simulink model "Lightning_McSeas_VCU_Current_Mode"  (R2021b)
settings: Solver=FixedStepDiscrete  StartTime=0.0  StopTime=10.0  FixedStep=0.01  RelTol=1e-3  EnableMultiTasking=on
PreLoadFcn:
  | try, model_open; catch, disp('Error occurred while executing model pre-load callback: model_open.m'); disp('Please assure that the MATLAB working directory is set to the model directory before opening.'); end
InitFcn:
  | try, model_open; catch, end
undefined symbols (not defined in the file): dataName, enumName, enumValue, GCM, raptor_get_safe_string
libraries: Raptor_lib x72, simulink x8
(part 3 of 3)

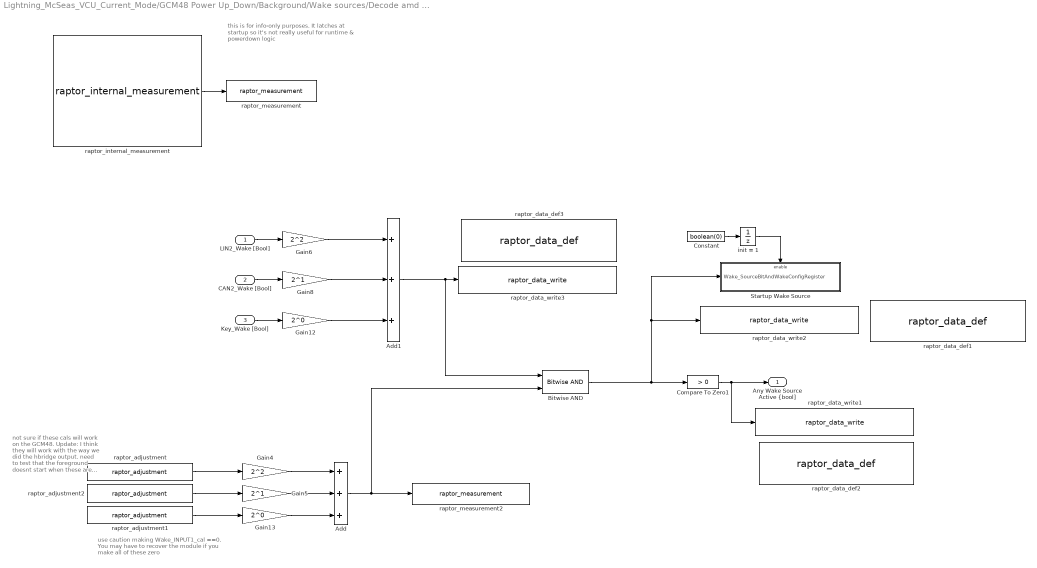
== system Lightning_McSeas_VCU_Current_Mode/GCM48 Power Up_Down/Background/Wake sources/Decode amd Ignore Some Wake Sources ==
  note: this is for info-only purposes. It latches at startup so it's not really useful for runtime & powerdown logic
  note: not sure if these cals will work on the GCM48. Update: I think they will work with the way we did the hbridge output. need to test that the foreground doesnt start when these are zero
  note: use caution making Wake_INPUT1_cal ==0. You may have to recover the module if you make all of these zero
  LIN2_Wake [Bool] : Inport
  CAN2_Wake [Bool] : Inport  Port=2
  Key_Wake [Bool] : Inport  Port=3
  Add : Sum  Inputs=3  OutDataTypeStr=uint16
  Add1 : Sum  Inputs=3  OutDataTypeStr=uint16
  Bitwise AND : simulink/Logic and Bit Operations/Bitwise Operator  logicop=AND  UseBitMask=off  NumInputPorts=2  BitMask=bin2dec('11011001')  BitMaskRealWorld=Stored Integer
  Compare To Zero1 : simulink/Logic and Bit Operations/Compare To Zero  relop=>  OutDataTypeStr=boolean
  Constant : Constant  Value=boolean(0)
  Gain12 : Gain  Gain=2^0  OutDataTypeStr=uint16
  Gain13 : Gain  Gain=2^0  OutDataTypeStr=uint16
  Gain4 : Gain  Gain=2^2  OutDataTypeStr=uint16
  Gain5 : Gain  Gain=2^1  OutDataTypeStr=uint16
  Gain6 : Gain  Gain=2^2  OutDataTypeStr=uint16
  Gain8 : Gain  Gain=2^1  OutDataTypeStr=uint16
  Startup Wake Source : Subsystem  TreatAsAtomicUnit=on
  init = 1 : UnitDelay  InitialCondition=1  SampleTime=-1  HasFrameUpgradeWarning=on
  raptor_adjustment : Raptor_lib/Data Storage/raptor_adjustment  paramName='GCM48Wake_LIN2_cal'  nameSource=Parameter  initValue=0  dataType=boolean  storage=Calibration  calDispType=Number  calEnum={'False', 'True'}  calGain=1.0  calOffset=0.0  calMax=inf  calMin=-inf  calFormat='-1'  calUnit='bool'  calHelp='1 configures the module to wake via this input, 0 ignores this input'  calAccess=4  calFunction=group  calDispHeaders=off  calColHeaders={'Col1' 'Col2' 'Col3'}  calRowHeaders={'Row1' 'Row2' 'Row3'}
      settings: SourceProductName=Raptor
  raptor_adjustment1 : Raptor_lib/Data Storage/raptor_adjustment  paramName='GCM48Wake_INPUT1_cal'  nameSource=Parameter  initValue=1  dataType=boolean  storage=Calibration  calDispType=Number  calEnum={'False', 'True'}  calGain=1.0  calOffset=0.0  calMax=inf  calMin=-inf  calFormat='-1'  calUnit='bool'  calHelp='1 configures the module to wake via this input, 0 ignores this input'  calAccess=4  calFunction=group  calDispHeaders=off  calColHeaders={'Col1' 'Col2' 'Col3'}  calRowHeaders={'Row1' 'Row2' 'Row3'}
      settings: SourceProductName=Raptor
  raptor_adjustment2 : Raptor_lib/Data Storage/raptor_adjustment  paramName='GCM48Wake_CAN2_cal'  nameSource=Parameter  initValue=0  dataType=boolean  storage=Calibration  calDispType=Number  calEnum={'False', 'True'}  calGain=1.0  calOffset=0.0  calMax=inf  calMin=-inf  calFormat='-1'  calUnit='bool'  calHelp='1 configures the module to wake via this input, 0 ignores this input'  calAccess=4  calFunction=group  calDispHeaders=off  calColHeaders={'Col1' 'Col2' 'Col3'}  calRowHeaders={'Row1' 'Row2' 'Row3'}
      settings: SourceProductName=Raptor
  raptor_data_def1 : Raptor_lib/Data Storage/raptor_data_def  dataName='Wake_SourceBitAndWakeConfigRegister'  initValue=0  dataType=uint16  storage=Volatile (RAM)  calVisible=on  calType=Measurement  calDispType=Number  calEnum={'False', 'True'}  calGain=1.0  calOffset=0  calMin=-inf  calMax=inf  calFormat='-1'  calUnit=''  calHelp=''  calAccess=2  calFunction=group  calDispHeaders=off  calColHeaders={'Col1' 'Col2' 'Col3'}  calRowHeaders={'Row1' 'Row2' 'Row3'}
      settings: SourceProductName=Raptor
  raptor_data_def2 : Raptor_lib/Data Storage/raptor_data_def  dataName='Wake_AnyWakeSourceActive'  initValue=0  dataType=boolean  storage=Volatile (RAM)  calVisible=on  calType=Measurement  calDispType=Number  calEnum={'False', 'True'}  calGain=1.0  calOffset=0  calMin=-inf  calMax=inf  calFormat='-1'  calUnit='any wake source is keeping the module alive'  calHelp='bool'  calAccess=2  calFunction=group  calDispHeaders=off  calColHeaders={'Col1' 'Col2' 'Col3'}  calRowHeaders={'Row1' 'Row2' 'Row3'}
      settings: SourceProductName=Raptor
  raptor_data_def3 : Raptor_lib/Data Storage/raptor_data_def  dataName='WakeSource_Current'  initValue=0  dataType=uint16  storage=Volatile (RAM)  calVisible=on  calType=Measurement  calDispType=Number  calEnum={'False', 'True'}  calGain=1.0  calOffset=0  calMin=-inf  calMax=inf  calFormat='-1'  calUnit='wake source at the current instant'  calHelp=''  calAccess=2  calFunction=group  calDispHeaders=off  calColHeaders={'Col1' 'Col2' 'Col3'}  calRowHeaders={'Row1' 'Row2' 'Row3'}
      settings: SourceProductName=Raptor
  raptor_data_write1 : Raptor_lib/Data Storage/raptor_data_write  dataName='Wake_AnyWakeSourceActive'  dataShape=Scalar  idxSource=Input Port  idxRow=1  idxCol=1
      settings: SourceProductName=Raptor
  raptor_data_write2 : Raptor_lib/Data Storage/raptor_data_write  dataName='Wake_SourceBitAndWakeConfigRegister'  dataShape=Scalar  idxSource=Input Port  idxRow=1  idxCol=1
      settings: SourceProductName=Raptor
  raptor_data_write3 : Raptor_lib/Data Storage/raptor_data_write  dataName='WakeSource_Current'  dataShape=Scalar  idxSource=Input Port  idxRow=1  idxCol=1
      settings: SourceProductName=Raptor
  raptor_internal_measurement : Raptor_lib/Input & Output/raptor_internal_measurement  resourceValues=OUTPUT1_VFB|OUTPUT2_VFB|OUTPUT3_VFB|OUTPUT4_VFB|OUTPUT5_VFB|OUTPUT6_VFB|OUTPUT7_VFB|OUTPUT8_VFB|OUTPUT11_VFB|OUTPUT12_VFB|OUTPUT13_VFB|OUTPUT14_VFB|OUTPUT15_VFB|OUTPUT2_DFB|OUTPUT3_DFB|HBRIDGE9_10_DFB|OUTPUT2_IFB|OUTPUT3_IFB|HBRIDGE9_10_IFB|SENS_SUPPLY1_VFB|SENS_SUPPLY2_VFB|NTC_TEMP|WAKE_SOURCE|(None)  resource=WAKE_SOURCE  out_eng=0  soft_filter=1  out_bool=0
      settings: SourceProductName=Raptor
  raptor_measurement : Raptor_lib/Data Storage/raptor_measurement  paramName='WakeSource_RaptorIntrnlMeas'  nameSource=Parameter  calDispType=Number  calEnum={'False', 'True'}  calGain=1.0  calOffset=0.0  calMax=inf  calMin=-inf  calFormat='-1'  calUnit='wake source at startup... kinda. it often reads that LIN work the module even if the LIN bus isnt connected.'  calHelp=''  calAccess=4  calFunction=group  calVisible=on
      settings: SourceProductName=Raptor
  raptor_measurement2 : Raptor_lib/Data Storage/raptor_measurement  paramName='WakeConfigRegister'  nameSource=Parameter  calDispType=Number  calEnum={'False', 'True'}  calGain=1.0  calOffset=0.0  calMax=inf  calMin=-inf  calFormat='-1'  calUnit='register'  calHelp=''  calAccess=4  calFunction=group  calVisible=on
      settings: SourceProductName=Raptor
  "Any Wake Source Active {bool]" : Outport  VectorParamsAs1DForOutWhenUnconnected=off
  wires:
  Key_Wake [Bool]/1 -> Gain12/1
  init = 1/1 -> Startup Wake Source/Enable
  Constant/1 -> init = 1/1
  Compare To Zero1/1 -> "Any Wake Source Active {bool]"/1, raptor_data_write1/1
  LIN2_Wake [Bool]/1 -> Gain6/1
  CAN2_Wake [Bool]/1 -> Gain8/1
  raptor_adjustment1/1 -> Gain13/1
  Gain13/1 -> Add/3
  Gain12/1 -> Add1/3
  Add1/1 -> raptor_data_write3/1, Bitwise AND/1
  Gain6/1 -> Add1/1
  Gain8/1 -> Add1/2
  Bitwise AND/1 -> raptor_data_write2/1, Startup Wake Source/1(Wake_SourceBitAndWakeConfigRegister), Compare To Zero1/1
  raptor_adjustment2/1 -> Gain5/1
  Gain5/1 -> Add/2
  Add/1 -> raptor_measurement2/1, Bitwise AND/2
  raptor_internal_measurement/1 -> raptor_measurement/1
  raptor_adjustment/1 -> Gain4/1
  Gain4/1 -> Add/1

== system Lightning_McSeas_VCU_Current_Mode/GCM48 Power Up_Down/Background/Wake sources/Dtc ==
  In : Inport
  Delay Input1 : UnitDelay  Description=Store in Global RAM  DisableCoverage=on  InitialCondition=init  SampleTime=-1  HasFrameUpgradeWarning=on
  Relational Operator : RelationalOperator  Operator===  OutDataTypeStr=boolean  RndMeth=Nearest  InputSameDT=on
  Bool : Outport  InitialOutput=0  VectorParamsAs1DForOutWhenUnconnected=off
  wires:
  In/1 -> Delay Input1/1, Relational Operator/1
  Delay Input1/1 -> Relational Operator/2
  Relational Operator/1 -> Bool/1

== system Lightning_McSeas_VCU_Current_Mode/GCM48 Power Up_Down/Background/Wake sources/Dtc1 ==
  In : Inport
  Delay Input1 : UnitDelay  Description=Store in Global RAM  DisableCoverage=on  InitialCondition=init  SampleTime=-1  HasFrameUpgradeWarning=on
  Relational Operator : RelationalOperator  Operator===  OutDataTypeStr=boolean  RndMeth=Nearest  InputSameDT=on
  Bool : Outport  InitialOutput=0  VectorParamsAs1DForOutWhenUnconnected=off
  wires:
  Relational Operator/1 -> Bool/1
  Delay Input1/1 -> Relational Operator/2
  In/1 -> Relational Operator/1, Delay Input1/1

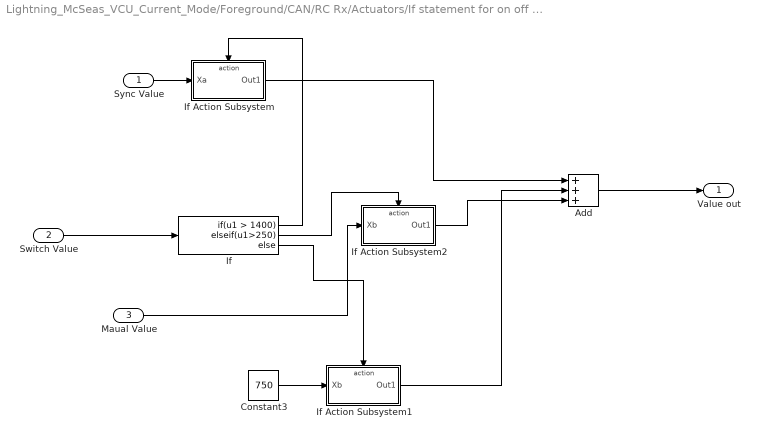
== system Lightning_McSeas_VCU_Current_Mode/Foreground/CAN/RC Rx/Actuators/If statement for on off switch1 ==
  Sync Value : Inport
  Switch Value : Inport  Port=2
  Maual Value : Inport  Port=3
  Add : Sum  Inputs=+++
  Constant3 : Constant  Value=750
  If : If  IfExpression=u1 > 1400  ElseIfExpressions=u1>250
  If Action Subsystem : Subsystem  TreatAsAtomicUnit=on
  If Action Subsystem1 : Subsystem  TreatAsAtomicUnit=on
  If Action Subsystem2 : Subsystem  TreatAsAtomicUnit=on
  Value out : Outport
  wires:
  If/3 -> If Action Subsystem1/Action
  Switch Value/1 -> If/1
  Sync Value/1 -> If Action Subsystem/1(Xa)
  If Action Subsystem1/1(Out1) -> Add/2
  Add/1 -> Value out/1
  If/1 -> If Action Subsystem/Action
  Constant3/1 -> If Action Subsystem1/1(Xb)
  If Action Subsystem/1(Out1) -> Add/1
  If/2 -> If Action Subsystem2/Action
  If Action Subsystem2/1(Out1) -> Add/3
  Maual Value/1 -> If Action Subsystem2/1(Xb)

== system Lightning_McSeas_VCU_Current_Mode/Foreground/CAN/RC Rx/Actuators/Subsystem ==
  Front left : Inport
  Rise of Front : Inport  Port=2
  Gain : Gain  Gain=1/1500
  Product : Product
  Actuator value : Outport
  wires:
  Front left/1 -> Gain/1
  Rise of Front/1 -> Product/1
  Gain/1 -> Product/2
  Product/1 -> Actuator value/1

== system Lightning_McSeas_VCU_Current_Mode/Foreground/CAN/RC Rx/Battery Charging/Max Voltage Cell Control ==
  note: 0 = Charging
      | 1 = STOP
  In1 : Inport
  Constant : Constant  Value=0
  Constant1 : Constant
  If : If  IfExpression=u1 > 4.15
  If Action Subsystem : Subsystem  TreatAsAtomicUnit=on
  If Action Subsystem1 : Subsystem  TreatAsAtomicUnit=on
  Merge : Merge
  Out1 : Outport
  wires:
  In1/1 -> If/1
  If/1 -> If Action Subsystem/Action
  If/2 -> If Action Subsystem1/Action
  Constant/1 -> If Action Subsystem/1(In1)
  Constant1/1 -> If Action Subsystem1/1(In1)
  If Action Subsystem/1(Out1) -> Merge/1
  If Action Subsystem1/1(Out1) -> Merge/2
  Merge/1 -> Out1/1

== system Lightning_McSeas_VCU_Current_Mode/Foreground/CAN/RC Rx/Battery Charging/Subsystem1 ==
  In1 : Inport
  In2 : Inport  Port=2
  Constant : Constant  Value=16
  Constant1 : Constant  Value=3.9
  If : If  IfExpression=u1 < 4.05  ElseIfExpressions=u1 < 4.10
  If Action Subsystem : Subsystem  TreatAsAtomicUnit=on
  If Action Subsystem1 : Subsystem  TreatAsAtomicUnit=on
  If Action Subsystem2 : Subsystem  TreatAsAtomicUnit=on
  Merge : Merge  Inputs=3
  Out1 : Outport
  wires:
  In1/1 -> If/1
  If/1 -> If Action Subsystem/Action
  If/3 -> If Action Subsystem1/Action
  Constant/1 -> If Action Subsystem/1(In1)
  Constant1/1 -> If Action Subsystem1/1(In1)
  If Action Subsystem/1(Out1) -> Merge/1
  If Action Subsystem1/1(Out1) -> Merge/3
  Merge/1 -> Out1/1
  If/2 -> If Action Subsystem2/Action
  In2/1 -> If Action Subsystem2/1(In1)
  If Action Subsystem2/1(Out1) -> Merge/2

== system Lightning_McSeas_VCU_Current_Mode/Foreground/CAN/RC Rx/Battery Charging/Switch Control ==
  note: 0 = Charging
      | 1 = STOP
  In1 : Inport
  Constant : Constant  Value=0
  Constant1 : Constant
  If : If  IfExpression=u1 > 1200
  If Action Subsystem : Subsystem  TreatAsAtomicUnit=on
  If Action Subsystem1 : Subsystem  TreatAsAtomicUnit=on
  Merge : Merge
  Out1 : Outport
  wires:
  In1/1 -> If/1
  If/1 -> If Action Subsystem/Action
  If/2 -> If Action Subsystem1/Action
  Constant/1 -> If Action Subsystem/1(In1)
  Constant1/1 -> If Action Subsystem1/1(In1)
  If Action Subsystem/1(Out1) -> Merge/1
  If Action Subsystem1/1(Out1) -> Merge/2
  Merge/1 -> Out1/1

== system Lightning_McSeas_VCU_Current_Mode/Foreground/CAN/RC Rx/Battery Switch/If statement for on off switch ==
  value in : Inport
  Constant2 : Constant
  Constant3 : Constant  Value=0
  If : If  IfExpression=u1 > 1200
  If Action Subsystem : Subsystem  TreatAsAtomicUnit=on
  If Action Subsystem1 : Subsystem  TreatAsAtomicUnit=on
  Merge : Merge
  Value out : Outport
  wires:
  If/2 -> If Action Subsystem1/Action
  value in/1 -> If/1
  Constant2/1 -> If Action Subsystem/1(Xa)
  If Action Subsystem1/1(Out1) -> Merge/2
  Merge/1 -> Value out/1
  If/1 -> If Action Subsystem/Action
  Constant3/1 -> If Action Subsystem1/1(Xb)
  If Action Subsystem/1(Out1) -> Merge/1

== system Lightning_McSeas_VCU_Current_Mode/Foreground/CAN/RC Rx/Battery Switch/If statement for on off switch1 ==
  value in : Inport
  Constant2 : Constant  OutDataTypeStr=boolean
  Constant3 : Constant  Value=0  OutDataTypeStr=boolean
  If : If  IfExpression=u1 > 1200
  If Action Subsystem : Subsystem  TreatAsAtomicUnit=on
  If Action Subsystem1 : Subsystem  TreatAsAtomicUnit=on
  Merge : Merge
  Value out : Outport
  wires:
  value in/1 -> If/1
  Constant2/1 -> If Action Subsystem/1(Xa)
  If Action Subsystem1/1(Out1) -> Merge/2
  Merge/1 -> Value out/1
  If/1 -> If Action Subsystem/Action
  Constant3/1 -> If Action Subsystem1/1(Xb)
  If Action Subsystem/1(Out1) -> Merge/1
  If/2 -> If Action Subsystem1/Action

== system Lightning_McSeas_VCU_Current_Mode/Foreground/CAN/RC Rx/Battery Switch/If statement for on off switch2 ==
  value in : Inport
  Constant2 : Constant
  Constant3 : Constant  Value=0
  If : If  IfExpression=u1 > 250
  If Action Subsystem : Subsystem  TreatAsAtomicUnit=on
  If Action Subsystem1 : Subsystem  TreatAsAtomicUnit=on
  Merge : Merge
  Value out : Outport
  wires:
  If/2 -> If Action Subsystem1/Action
  value in/1 -> If/1
  Constant2/1 -> If Action Subsystem/1(Xa)
  If Action Subsystem1/1(Out1) -> Merge/2
  Merge/1 -> Value out/1
  If/1 -> If Action Subsystem/Action
  Constant3/1 -> If Action Subsystem1/1(Xb)
  If Action Subsystem/1(Out1) -> Merge/1

== system Lightning_McSeas_VCU_Current_Mode/Foreground/CAN/RC Rx/MCU/If statement for on off switch1 ==
  value in : Inport
  Constant2 : Constant
  Constant3 : Constant  Value=0
  If : If  IfExpression=u1 > 1200
  If Action Subsystem : Subsystem  TreatAsAtomicUnit=on
  If Action Subsystem1 : Subsystem  TreatAsAtomicUnit=on
  Merge : Merge
  Value out : Outport
  wires:
  value in/1 -> If/1
  Constant2/1 -> If Action Subsystem/1(Xa)
  If Action Subsystem1/1(Out1) -> Merge/2
  Merge/1 -> Value out/1
  If/1 -> If Action Subsystem/Action
  Constant3/1 -> If Action Subsystem1/1(Xb)
  If Action Subsystem/1(Out1) -> Merge/1
  If/2 -> If Action Subsystem1/Action

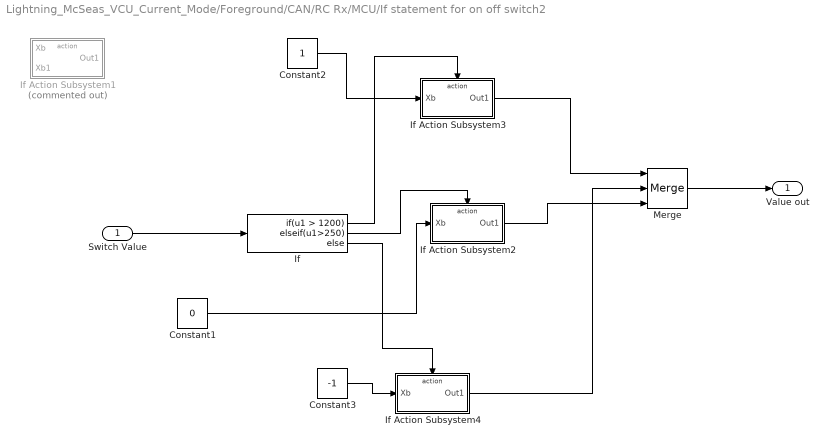
== system Lightning_McSeas_VCU_Current_Mode/Foreground/CAN/RC Rx/MCU/If statement for on off switch2 ==
  Switch Value : Inport
  Constant1 : Constant  Value=0
  Constant2 : Constant
  Constant3 : Constant  Value=-1
  If : If  IfExpression=u1 > 1200  ElseIfExpressions=u1>250
  If Action Subsystem1 : Subsystem  Commented=on  TreatAsAtomicUnit=on
  If Action Subsystem2 : Subsystem  TreatAsAtomicUnit=on
  If Action Subsystem3 : Subsystem  TreatAsAtomicUnit=on
  If Action Subsystem4 : Subsystem  TreatAsAtomicUnit=on
  Merge : Merge  Inputs=3
  Value out : Outport
  wires:
  If/3 -> If Action Subsystem4/Action
  Switch Value/1 -> If/1
  If Action Subsystem4/1(Out1) -> Merge/2
  Merge/1 -> Value out/1
  Constant3/1 -> If Action Subsystem4/1(Xb)
  If/2 -> If Action Subsystem2/Action
  If Action Subsystem2/1(Out1) -> Merge/3
  Constant1/1 -> If Action Subsystem2/1(Xb)
  Constant2/1 -> If Action Subsystem3/1(Xb)
  If Action Subsystem3/1(Out1) -> Merge/1
  If/1 -> If Action Subsystem3/Action

== system Lightning_McSeas_VCU_Current_Mode/Foreground/CAN/RC Rx/MCU/If statement for on off switch3 ==
  Switch Value : Inport
  Add : Sum  Inputs=+++
  Constant1 : Constant  Value=0
  Constant2 : Constant
  Constant3 : Constant  Value=-1
  If : If  IfExpression=u1 > 1200  ElseIfExpressions=u1>250
  If Action Subsystem1 : Subsystem  TreatAsAtomicUnit=on
  If Action Subsystem2 : Subsystem  TreatAsAtomicUnit=on
  If Action Subsystem3 : Subsystem  TreatAsAtomicUnit=on
  Value out : Outport
  wires:
  If/3 -> If Action Subsystem1/Action
  Switch Value/1 -> If Action Subsystem1/1(Xb), If Action Subsystem3/1(Xb), If/1
  If Action Subsystem1/1(Out1) -> Add/2
  Add/1 -> Value out/1
  Constant3/1 -> If Action Subsystem1/2(Xb1)
  If/2 -> If Action Subsystem2/Action
  If Action Subsystem2/1(Out1) -> Add/3
  Constant1/1 -> If Action Subsystem2/1(Xb)
  If/1 -> If Action Subsystem3/Action
  Constant2/1 -> If Action Subsystem3/2(Xb1)
  If Action Subsystem3/1(Out1) -> Add/1

== system Lightning_McSeas_VCU_Current_Mode/Foreground/CAN/RC Rx/MCU/If statement for on off switch4 ==
  value in : Inport
  Constant2 : Constant
  Constant3 : Constant  Value=0
  If : If  IfExpression=u1 >250
  If Action Subsystem : Subsystem  TreatAsAtomicUnit=on
  If Action Subsystem1 : Subsystem  TreatAsAtomicUnit=on
  Merge : Merge
  Value out : Outport
  wires:
  value in/1 -> If/1
  Constant2/1 -> If Action Subsystem/1(Xa)
  If Action Subsystem1/1(Out1) -> Merge/2
  Merge/1 -> Value out/1
  If/1 -> If Action Subsystem/Action
  Constant3/1 -> If Action Subsystem1/1(Xb)
  If Action Subsystem/1(Out1) -> Merge/1
  If/2 -> If Action Subsystem1/Action

== system Lightning_McSeas_VCU_Current_Mode/Foreground/CAN/RC Rx/MCU/If statement for on off switch5 ==
  Contact value : Inport
  Add : Sum
  If : If  IfExpression=u1 < 1
  If Action Subsystem1 : Subsystem  TreatAsAtomicUnit=on
  If Action Subsystem3 : Subsystem  TreatAsAtomicUnit=on
  Value out : Outport
  wires:
  If/2 -> If Action Subsystem1/Action
  Contact value/1 -> If Action Subsystem1/1(Xb1), If Action Subsystem3/1(Xb1), If/1
  If Action Subsystem1/1(Out1) -> Add/2
  Add/1 -> Value out/1
  If/1 -> If Action Subsystem3/Action
  If Action Subsystem3/1(Out1) -> Add/1

== system Lightning_McSeas_VCU_Current_Mode/Foreground/CAN/RC Rx/MCU/Left Motor ==
  Throttle : Inport
  Rudder : Inport  Port=2
  Drive Mode : Inport  Port=3
  If statement for on off switch1 : Subsystem
  Sum : Sum  Inputs=|+-
  Value out : Outport
  wires:
  Throttle/1 -> Sum/1
  Sum/1 -> If statement for on off switch1/2(Throttle)
  Rudder/1 -> Sum/2
  Drive Mode/1 -> If statement for on off switch1/1(Drive Mode swtich)
  If statement for on off switch1/1(Value out) -> Value out/1

== system Lightning_McSeas_VCU_Current_Mode/Foreground/CAN/RC Rx/MCU/Right Motor ==
  Throttle : Inport
  Rudder : Inport  Port=2
  Drive Mode : Inport  Port=3
  Constant : Constant  Value=-1
  If statement for on off switch1 : Subsystem
  Product : Product
  Sum : Sum  Inputs=|+-
  Value out : Outport
  wires:
  Throttle/1 -> Sum/1
  Sum/1 -> If statement for on off switch1/2(Throttle)
  Rudder/1 -> Sum/2
  Drive Mode/1 -> If statement for on off switch1/1(Drive Mode swtich)
  If statement for on off switch1/1(Value out) -> Product/1
  Product/1 -> Value out/1
  Constant/1 -> Product/2

== system Lightning_McSeas_VCU_Current_Mode/GCM48 Power Up_Down/Background/Wake sources/Debounce2/SetRst Init = 0 ==
  Set : Inport
  Rst : Inport  Port=2
  Constant : Constant  Value=boolean(0)
  Constant1 : Constant  Value=boolean(1)
  Multiport Switch : MultiPortSwitch  DataPortOrder=Zero-based contiguous  Inputs=2  zeroidx=on
  Multiport Switch1 : MultiPortSwitch  DataPortOrder=Zero-based contiguous  Inputs=2  zeroidx=on
  Unit Delay : UnitDelay  InitialCondition=init  SampleTime=-1  HasFrameUpgradeWarning=on
  Bool : Outport  VectorParamsAs1DForOutWhenUnconnected=off
  wires:
  Multiport Switch1/1 -> Multiport Switch/2
  Constant1/1 -> Multiport Switch1/3
  Constant/1 -> Multiport Switch/3
  Rst/1 -> Multiport Switch/1
  Set/1 -> Multiport Switch1/1
  Multiport Switch/1 -> Bool/1, Unit Delay/1
  Unit Delay/1 -> Multiport Switch1/2

== system Lightning_McSeas_VCU_Current_Mode/GCM48 Power Up_Down/Background/Wake sources/Decode amd Ignore Some Wake Sources/Startup Wake Source ==
  Wake_SourceBitAndWakeConfigRegister : Inport
  Enable : EnablePort
  raptor_measurement : Raptor_lib/Data Storage/raptor_measurement  paramName='WakeSource_Startup'  nameSource=Parameter  calDispType=Number  calEnum={'False', 'True'}  calGain=1.0  calOffset=0.0  calMax=inf  calMin=-inf  calFormat='-1'  calUnit=''  calHelp=''  calAccess=4  calFunction=group  calVisible=on
      settings: SourceProductName=Raptor
  wires:
  Wake_SourceBitAndWakeConfigRegister/1 -> raptor_measurement/1

== system Lightning_McSeas_VCU_Current_Mode/Foreground/CAN/RC Rx/Actuators/If statement for on off switch1/If Action Subsystem ==
  Xa : Inport
  Action Port : ActionPort
  Out1 : Outport
  wires:
  Xa/1 -> Out1/1

== system Lightning_McSeas_VCU_Current_Mode/Foreground/CAN/RC Rx/Actuators/If statement for on off switch1/If Action Subsystem1 ==
  Xb : Inport
  Action Port : ActionPort
  Out1 : Outport
  wires:
  Xb/1 -> Out1/1

== system Lightning_McSeas_VCU_Current_Mode/Foreground/CAN/RC Rx/Actuators/If statement for on off switch1/If Action Subsystem2 ==
  Xb : Inport
  Action Port : ActionPort
  Out1 : Outport
  wires:
  Xb/1 -> Out1/1

== system Lightning_McSeas_VCU_Current_Mode/Foreground/CAN/RC Rx/Battery Charging/Max Voltage Cell Control/If Action Subsystem ==
  In1 : Inport
  Action Port : ActionPort  ActionPortLabel=if(u1 > 4.15)
  Out1 : Outport
  wires:
  In1/1 -> Out1/1

== system Lightning_McSeas_VCU_Current_Mode/Foreground/CAN/RC Rx/Battery Charging/Max Voltage Cell Control/If Action Subsystem1 ==
  In1 : Inport
  Action Port : ActionPort  ActionPortLabel=else
  Out1 : Outport
  wires:
  In1/1 -> Out1/1

== system Lightning_McSeas_VCU_Current_Mode/Foreground/CAN/RC Rx/Battery Charging/Subsystem1/If Action Subsystem ==
  In1 : Inport
  Action Port : ActionPort  ActionPortLabel=if(u1 < 4.05)
  Out1 : Outport
  wires:
  In1/1 -> Out1/1

== system Lightning_McSeas_VCU_Current_Mode/Foreground/CAN/RC Rx/Battery Charging/Subsystem1/If Action Subsystem1 ==
  In1 : Inport
  Action Port : ActionPort  ActionPortLabel=else
  Out1 : Outport
  wires:
  In1/1 -> Out1/1

== system Lightning_McSeas_VCU_Current_Mode/Foreground/CAN/RC Rx/Battery Charging/Subsystem1/If Action Subsystem2 ==
  In1 : Inport
  Action Port : ActionPort  ActionPortLabel=elseif(u1 < 4.10)
  Out1 : Outport
  wires:
  In1/1 -> Out1/1

== system Lightning_McSeas_VCU_Current_Mode/Foreground/CAN/RC Rx/Battery Charging/Switch Control/If Action Subsystem ==
  In1 : Inport
  Action Port : ActionPort  ActionPortLabel=if(u1 > 1200)
  Out1 : Outport
  wires:
  In1/1 -> Out1/1

== system Lightning_McSeas_VCU_Current_Mode/Foreground/CAN/RC Rx/Battery Charging/Switch Control/If Action Subsystem1 ==
  In1 : Inport
  Action Port : ActionPort  ActionPortLabel=else
  Out1 : Outport
  wires:
  In1/1 -> Out1/1

== system Lightning_McSeas_VCU_Current_Mode/Foreground/CAN/RC Rx/Battery Switch/If statement for on off switch/If Action Subsystem ==
  Xa : Inport
  Action Port : ActionPort  ActionPortLabel=if(u1 > 1200)
  Out1 : Outport
  wires:
  Xa/1 -> Out1/1

== system Lightning_McSeas_VCU_Current_Mode/Foreground/CAN/RC Rx/Battery Switch/If statement for on off switch/If Action Subsystem1 ==
  Xb : Inport
  Action Port : ActionPort  ActionPortLabel=else
  Out1 : Outport
  wires:
  Xb/1 -> Out1/1

== system Lightning_McSeas_VCU_Current_Mode/Foreground/CAN/RC Rx/Battery Switch/If statement for on off switch1/If Action Subsystem ==
  Xa : Inport
  Action Port : ActionPort  ActionPortLabel=if(u1 > 1200)
  Out1 : Outport
  wires:
  Xa/1 -> Out1/1

== system Lightning_McSeas_VCU_Current_Mode/Foreground/CAN/RC Rx/Battery Switch/If statement for on off switch1/If Action Subsystem1 ==
  Xb : Inport
  Action Port : ActionPort  ActionPortLabel=else
  Out1 : Outport
  wires:
  Xb/1 -> Out1/1

== system Lightning_McSeas_VCU_Current_Mode/Foreground/CAN/RC Rx/Battery Switch/If statement for on off switch2/If Action Subsystem ==
  Xa : Inport
  Action Port : ActionPort  ActionPortLabel=if(u1 > 250)
  Out1 : Outport
  wires:
  Xa/1 -> Out1/1

== system Lightning_McSeas_VCU_Current_Mode/Foreground/CAN/RC Rx/Battery Switch/If statement for on off switch2/If Action Subsystem1 ==
  Xb : Inport
  Action Port : ActionPort  ActionPortLabel=else
  Out1 : Outport
  wires:
  Xb/1 -> Out1/1

== system Lightning_McSeas_VCU_Current_Mode/Foreground/CAN/RC Rx/MCU/If statement for on off switch1/If Action Subsystem ==
  Xa : Inport
  Action Port : ActionPort  ActionPortLabel=if(u1 > 1200)
  Out1 : Outport
  wires:
  Xa/1 -> Out1/1

== system Lightning_McSeas_VCU_Current_Mode/Foreground/CAN/RC Rx/MCU/If statement for on off switch1/If Action Subsystem1 ==
  Xb : Inport
  Action Port : ActionPort  ActionPortLabel=else
  Out1 : Outport
  wires:
  Xb/1 -> Out1/1

== system Lightning_McSeas_VCU_Current_Mode/Foreground/CAN/RC Rx/MCU/If statement for on off switch2/If Action Subsystem1 ==
  Xb : Inport
  Xb1 : Inport  Port=2
  Action Port : ActionPort
  Product : Product
  Out1 : Outport
  wires:
  Xb/1 -> Product/2
  Xb1/1 -> Product/1
  Product/1 -> Out1/1

== system Lightning_McSeas_VCU_Current_Mode/Foreground/CAN/RC Rx/MCU/If statement for on off switch2/If Action Subsystem2 ==
  Xb : Inport
  Action Port : ActionPort  ActionPortLabel=elseif(u1>250)
  Out1 : Outport
  wires:
  Xb/1 -> Out1/1

== system Lightning_McSeas_VCU_Current_Mode/Foreground/CAN/RC Rx/MCU/If statement for on off switch2/If Action Subsystem3 ==
  Xb : Inport
  Action Port : ActionPort  ActionPortLabel=if(u1 > 1200)
  Out1 : Outport
  wires:
  Xb/1 -> Out1/1

== system Lightning_McSeas_VCU_Current_Mode/Foreground/CAN/RC Rx/MCU/If statement for on off switch2/If Action Subsystem4 ==
  Xb : Inport
  Action Port : ActionPort  ActionPortLabel=else
  Out1 : Outport
  wires:
  Xb/1 -> Out1/1

== system Lightning_McSeas_VCU_Current_Mode/Foreground/CAN/RC Rx/MCU/If statement for on off switch3/If Action Subsystem1 ==
  Xb : Inport
  Xb1 : Inport  Port=2
  Action Port : ActionPort
  Product : Product
  Out1 : Outport
  wires:
  Xb/1 -> Product/2
  Xb1/1 -> Product/1
  Product/1 -> Out1/1

== system Lightning_McSeas_VCU_Current_Mode/Foreground/CAN/RC Rx/MCU/If statement for on off switch3/If Action Subsystem2 ==
  Xb : Inport
  Action Port : ActionPort
  Out1 : Outport
  wires:
  Xb/1 -> Out1/1

== system Lightning_McSeas_VCU_Current_Mode/Foreground/CAN/RC Rx/MCU/If statement for on off switch3/If Action Subsystem3 ==
  Xb : Inport
  Xb1 : Inport  Port=2
  Action Port : ActionPort
  Product : Product
  Out1 : Outport
  wires:
  Xb/1 -> Product/2
  Xb1/1 -> Product/1
  Product/1 -> Out1/1

== system Lightning_McSeas_VCU_Current_Mode/Foreground/CAN/RC Rx/MCU/If statement for on off switch4/If Action Subsystem ==
  Xa : Inport
  Action Port : ActionPort  ActionPortLabel=if(u1 >250)
  Out1 : Outport
  wires:
  Xa/1 -> Out1/1

== system Lightning_McSeas_VCU_Current_Mode/Foreground/CAN/RC Rx/MCU/If statement for on off switch4/If Action Subsystem1 ==
  Xb : Inport
  Action Port : ActionPort  ActionPortLabel=else
  Out1 : Outport
  wires:
  Xb/1 -> Out1/1

== system Lightning_McSeas_VCU_Current_Mode/Foreground/CAN/RC Rx/MCU/If statement for on off switch5/If Action Subsystem1 ==
  Xb1 : Inport
  Action Port : ActionPort
  Out1 : Outport
  wires:
  Xb1/1 -> Out1/1

== system Lightning_McSeas_VCU_Current_Mode/Foreground/CAN/RC Rx/MCU/If statement for on off switch5/If Action Subsystem3 ==
  Xb1 : Inport
  Action Port : ActionPort
  Transport Delay : TransportDelay  DelayTime=0.5
  Out1 : Outport
  wires:
  Xb1/1 -> Transport Delay/1
  Transport Delay/1 -> Out1/1

== system Lightning_McSeas_VCU_Current_Mode/Foreground/CAN/RC Rx/MCU/Left Motor/If statement for on off switch1 ==
  Drive Mode swtich : Inport
  Throttle : Inport  Port=2
  Add : Sum  Inputs=+++
  Constant3 : Constant  Value=0
  If : If  IfExpression=u1 > 1400  ElseIfExpressions=u1<250
  If Action Subsystem : Subsystem  TreatAsAtomicUnit=on
  If Action Subsystem1 : Subsystem  TreatAsAtomicUnit=on
  If Action Subsystem2 : Subsystem  TreatAsAtomicUnit=on
  Value out : Outport
  wires:
  If Action Subsystem1/1(Out1) -> Add/2
  Add/1 -> Value out/1
  If/1 -> If Action Subsystem/Action
  Constant3/1 -> If Action Subsystem1/1(Xb)
  If Action Subsystem/1(Out1) -> Add/1
  If/3 -> If Action Subsystem1/Action
  Drive Mode swtich/1 -> If/1
  If/2 -> If Action Subsystem2/Action
  If Action Subsystem2/1(Out1) -> Add/3
  Throttle/1 -> If Action Subsystem2/1(Xa), If Action Subsystem/1(Xa)

== system Lightning_McSeas_VCU_Current_Mode/Foreground/CAN/RC Rx/MCU/Right Motor/If statement for on off switch1 ==
  Drive Mode swtich : Inport
  Throttle : Inport  Port=2
  Add : Sum  Inputs=+++
  Constant3 : Constant  Value=0
  If : If  IfExpression=u1 > 1400  ElseIfExpressions=u1<250
  If Action Subsystem : Subsystem  TreatAsAtomicUnit=on
  If Action Subsystem1 : Subsystem  TreatAsAtomicUnit=on
  If Action Subsystem2 : Subsystem  TreatAsAtomicUnit=on
  Value out : Outport
  wires:
  If Action Subsystem1/1(Out1) -> Add/2
  Add/1 -> Value out/1
  If/1 -> If Action Subsystem/Action
  Constant3/1 -> If Action Subsystem1/1(Xb)
  If Action Subsystem/1(Out1) -> Add/1
  If/3 -> If Action Subsystem1/Action
  Drive Mode swtich/1 -> If/1
  If/2 -> If Action Subsystem2/Action
  If Action Subsystem2/1(Out1) -> Add/3
  Throttle/1 -> If Action Subsystem2/1(Xa), If Action Subsystem/1(Xa)

== system Lightning_McSeas_VCU_Current_Mode/Foreground/CAN/RC Rx/MCU/Left Motor/If statement for on off switch1/If Action Subsystem ==
  Xa : Inport
  Action Port : ActionPort  ActionPortLabel=if(u1 > 1400)
  Out1 : Outport
  wires:
  Xa/1 -> Out1/1

== system Lightning_McSeas_VCU_Current_Mode/Foreground/CAN/RC Rx/MCU/Left Motor/If statement for on off switch1/If Action Subsystem1 ==
  Xb : Inport
  Action Port : ActionPort  ActionPortLabel=else
  Out1 : Outport
  wires:
  Xb/1 -> Out1/1

== system Lightning_McSeas_VCU_Current_Mode/Foreground/CAN/RC Rx/MCU/Left Motor/If statement for on off switch1/If Action Subsystem2 ==
  Xa : Inport
  Action Port : ActionPort  ActionPortLabel=elseif(u1<250)
  Constant : Constant  Value=-1
  Product : Product
  Out1 : Outport
  wires:
  Xa/1 -> Product/1
  Product/1 -> Out1/1
  Constant/1 -> Product/2

== system Lightning_McSeas_VCU_Current_Mode/Foreground/CAN/RC Rx/MCU/Right Motor/If statement for on off switch1/If Action Subsystem ==
  Xa : Inport
  Action Port : ActionPort  ActionPortLabel=if(u1 > 1400)
  Out1 : Outport
  wires:
  Xa/1 -> Out1/1

== system Lightning_McSeas_VCU_Current_Mode/Foreground/CAN/RC Rx/MCU/Right Motor/If statement for on off switch1/If Action Subsystem1 ==
  Xb : Inport
  Action Port : ActionPort  ActionPortLabel=else
  Out1 : Outport
  wires:
  Xb/1 -> Out1/1

== system Lightning_McSeas_VCU_Current_Mode/Foreground/CAN/RC Rx/MCU/Right Motor/If statement for on off switch1/If Action Subsystem2 ==
  Xa : Inport
  Action Port : ActionPort  ActionPortLabel=elseif(u1<250)
  Constant : Constant  Value=-1
  Product : Product
  Out1 : Outport
  wires:
  Xa/1 -> Product/1
  Product/1 -> Out1/1
  Constant/1 -> Product/2
